simulink model "IEEE30_case"  (R2024b)
settings: Solver=FixedStepAuto  StartTime=0  StopTime=5  FixedStep=1e-7  RelTol=1e-3
values from neighbouring files (symbols this model uses):
  GFL_DFIG_7_C_bus = 0.08    [IEEE30_case_parameters.m]
  GFL_DFIG_7_D_mutual = 2.500000e+3    (= 2500)    [IEEE30_case_parameters.m]
  GFL_DFIG_7_f0 = 60    [IEEE30_case_parameters.m]
  GFL_DFIG_7_gPLLi = 3200    [IEEE30_case_parameters.m]
  GFL_DFIG_7_gPLLp = 650    [IEEE30_case_parameters.m]
  GFL_DFIG_7_H_WT = 0.4    [IEEE30_case_parameters.m]
  GFL_DFIG_7_Hg = 0.8    [IEEE30_case_parameters.m]
  GFL_DFIG_7_Igq_ref = 0    [IEEE30_case_parameters.m]
  GFL_DFIG_7_Ird_ref = 704.45696    [IEEE30_case_parameters.m]
  GFL_DFIG_7_KI_V = -300000    [IEEE30_case_parameters.m]
  GFL_DFIG_7_KP_V = -1000    [IEEE30_case_parameters.m]
  GFL_DFIG_7_Ksh = 1.254300e+4    (= 12543)    [IEEE30_case_parameters.m]
  GFL_DFIG_7_Lg = 0.000483    [IEEE30_case_parameters.m]
  GFL_DFIG_7_Lm_pu = 4    [IEEE30_case_parameters.m]
  GFL_DFIG_7_N = 100    [IEEE30_case_parameters.m]
  GFL_DFIG_7_p = 2    [IEEE30_case_parameters.m]
  GFL_DFIG_7_Pitch = 0    [IEEE30_case_parameters.m]
  GFL_DFIG_7_R = 44    [IEEE30_case_parameters.m]
  GFL_DFIG_7_Rg = 2.000000e-5    (= 2e-05)    [IEEE30_case_parameters.m]
  GFL_DFIG_7_rho = 1.225    [IEEE30_case_parameters.m]
  GFL_DFIG_7_rPLLi = 4500    [IEEE30_case_parameters.m]
  GFL_DFIG_7_rPLLp = 620    [IEEE30_case_parameters.m]
  GFL_DFIG_7_Rs_pu = 0.011    [IEEE30_case_parameters.m]
  GFL_DFIG_7_Sbase = 2.000000e+6    (= 2000000)    [IEEE30_case_parameters.m]
  GFL_DFIG_7_ugq_ref = 0    [IEEE30_case_parameters.m]
  GFL_DFIG_7_usd_ref = 0    [IEEE30_case_parameters.m]
  GFL_DFIG_7_Vbase = 690    [IEEE30_case_parameters.m]
  GFL_DFIG_7_Vdc_ref = 1200    [IEEE30_case_parameters.m]
  GFL_DFIG_7_wind = 12    [IEEE30_case_parameters.m]
  GFL_DFIG_7_wm_ref = 518.184209    [IEEE30_case_parameters.m]
  SG_D_13_D = 0.01056    [IEEE30_case_parameters.m]
  SG_D_13_EnableSaturation = 0    [IEEE30_case_parameters.m]
  SG_D_13_f0 = 60    [IEEE30_case_parameters.m]
  SG_D_13_H = 7.5    [IEEE30_case_parameters.m]
  SG_D_13_K_A = 20    [IEEE30_case_parameters.m]
  SG_D_13_K_E = 1.000000e+1    (= 10)    [IEEE30_case_parameters.m]
  SG_D_13_K_F = 2.363    [IEEE30_case_parameters.m]
  SG_D_13_K_s = 0.5    [IEEE30_case_parameters.m]
  SG_D_13_R_a = 0.001088    [IEEE30_case_parameters.m]
  SG_D_13_S_A = 1    [IEEE30_case_parameters.m]
  SG_D_13_S_B = 0.103    [IEEE30_case_parameters.m]
  SG_D_13_S_N = 10.659857    [IEEE30_case_parameters.m]
  SG_D_13_SpeedPara = 200    [IEEE30_case_parameters.m]
  SG_D_13_T_0 = 0.370163    [IEEE30_case_parameters.m]
  SG_D_13_T_1 = 0.3    [IEEE30_case_parameters.m]
  SG_D_13_T_2 = 0.05    [IEEE30_case_parameters.m]
  SG_D_13_T_3 = 0.02    [IEEE30_case_parameters.m]
  SG_D_13_T_4 = 0.005    [IEEE30_case_parameters.m]
  SG_D_13_T_A = 0.02    [IEEE30_case_parameters.m]
  SG_D_13_T_dd = 8.000000e+0    (= 8)    [IEEE30_case_parameters.m]
  SG_D_13_T_ddd = 0.04    [IEEE30_case_parameters.m]
  SG_D_13_T_E = 0.314    [IEEE30_case_parameters.m]
  SG_D_13_T_F = 0.35    [IEEE30_case_parameters.m]
  SG_D_13_T_qd = 0.8    [IEEE30_case_parameters.m]
  SG_D_13_T_qdd = 0.02    [IEEE30_case_parameters.m]
  SG_D_13_T_speed = 0.1    [IEEE30_case_parameters.m]
  SG_D_13_T_w = 0.5    [IEEE30_case_parameters.m]
  SG_D_13_V_ref = 1.696619    [IEEE30_case_parameters.m]
  SG_D_13_w_ref = 376.991118    [IEEE30_case_parameters.m]
  SG_D_13_x_d = 1.9    [IEEE30_case_parameters.m]
  SG_D_13_x_dd = 0.302    [IEEE30_case_parameters.m]
  SG_D_13_x_ddd = 0.204    [IEEE30_case_parameters.m]
  SG_D_13_x_l = 0.05    [IEEE30_case_parameters.m]
  SG_D_13_x_q = 1.3    [IEEE30_case_parameters.m]
  SG_D_13_x_qd = 0.5    [IEEE30_case_parameters.m]
  SG_D_13_x_qdd = 0.3    [IEEE30_case_parameters.m]
  SG_D_1_D = 0.01056    [IEEE30_case_parameters.m]
  SG_D_1_EnableSaturation = 0    [IEEE30_case_parameters.m]
  SG_D_1_f0 = 60    [IEEE30_case_parameters.m]
  SG_D_1_H = 7.5    [IEEE30_case_parameters.m]
  SG_D_1_K_A = 20    [IEEE30_case_parameters.m]
  SG_D_1_K_E = 1.000000e+1    (= 10)    [IEEE30_case_parameters.m]
  SG_D_1_K_F = 2.363    [IEEE30_case_parameters.m]
  SG_D_1_K_s = 0.5    [IEEE30_case_parameters.m]
  SG_D_1_R_a = 0.001088    [IEEE30_case_parameters.m]
  SG_D_1_S_A = 1    [IEEE30_case_parameters.m]
  SG_D_1_S_B = 0.103    [IEEE30_case_parameters.m]
  SG_D_1_S_N = 10.659857    [IEEE30_case_parameters.m]
  SG_D_1_SpeedPara = 200    [IEEE30_case_parameters.m]
  SG_D_1_T_0 = 0.259812    [IEEE30_case_parameters.m]
  SG_D_1_T_1 = 0.3    [IEEE30_case_parameters.m]
  SG_D_1_T_2 = 0.05    [IEEE30_case_parameters.m]
  SG_D_1_T_3 = 0.02    [IEEE30_case_parameters.m]
  SG_D_1_T_4 = 0.005    [IEEE30_case_parameters.m]
  SG_D_1_T_A = 0.02    [IEEE30_case_parameters.m]
  SG_D_1_T_dd = 8.000000e+0    (= 8)    [IEEE30_case_parameters.m]
  SG_D_1_T_ddd = 0.04    [IEEE30_case_parameters.m]
  SG_D_1_T_E = 0.314    [IEEE30_case_parameters.m]
  SG_D_1_T_F = 0.35    [IEEE30_case_parameters.m]
  SG_D_1_T_qd = 0.8    [IEEE30_case_parameters.m]
  SG_D_1_T_qdd = 0.02    [IEEE30_case_parameters.m]
  SG_D_1_T_speed = 0.1    [IEEE30_case_parameters.m]
  SG_D_1_T_w = 0.5    [IEEE30_case_parameters.m]
  SG_D_1_V_ref = 1.544107    [IEEE30_case_parameters.m]
  SG_D_1_w_ref = 376.991118    [IEEE30_case_parameters.m]
  SG_D_1_x_d = 1.9    [IEEE30_case_parameters.m]
  SG_D_1_x_dd = 0.302    [IEEE30_case_parameters.m]
  SG_D_1_x_ddd = 0.204    [IEEE30_case_parameters.m]
  SG_D_1_x_l = 0.05    [IEEE30_case_parameters.m]
  SG_D_1_x_q = 1.3    [IEEE30_case_parameters.m]
  SG_D_1_x_qd = 0.5    [IEEE30_case_parameters.m]
  SG_D_1_x_qdd = 0.3    [IEEE30_case_parameters.m]
  SG_D_22_D = 0.01056    [IEEE30_case_parameters.m]
  SG_D_22_EnableSaturation = 0    [IEEE30_case_parameters.m]
  SG_D_22_f0 = 60    [IEEE30_case_parameters.m]
  SG_D_22_H = 7.5    [IEEE30_case_parameters.m]
  SG_D_22_K_A = 20    [IEEE30_case_parameters.m]
  SG_D_22_K_E = 1.000000e+1    (= 10)    [IEEE30_case_parameters.m]
  SG_D_22_K_F = 2.363    [IEEE30_case_parameters.m]
  SG_D_22_K_s = 0.5    [IEEE30_case_parameters.m]
  SG_D_22_R_a = 0.001088    [IEEE30_case_parameters.m]
  SG_D_22_S_A = 1    [IEEE30_case_parameters.m]
  SG_D_22_S_B = 0.103    [IEEE30_case_parameters.m]
  SG_D_22_S_N = 10.659857    [IEEE30_case_parameters.m]
  SG_D_22_SpeedPara = 200    [IEEE30_case_parameters.m]
  SG_D_22_T_0 = 0.216121    [IEEE30_case_parameters.m]
  SG_D_22_T_1 = 0.3    [IEEE30_case_parameters.m]
  SG_D_22_T_2 = 0.05    [IEEE30_case_parameters.m]
  SG_D_22_T_3 = 0.02    [IEEE30_case_parameters.m]
  SG_D_22_T_4 = 0.005    [IEEE30_case_parameters.m]
  ... (+126 more)
(part 18 of 27)

== system IEEE30_case/SG_D_13/d_R_f_SG_D_13_block ==
  note: d_R_f_SG_D_13 in IEEE30_case
      | $-\frac{R_{f,\mathrm{SG},D,13}-\frac{E_{\mathrm{fd},\mathrm{SG},D,13}\,K_{F}}{T_{F}}}{T_{F}}$
      | Automatically generated on 2025-11-01 18:35:19 .
  State_E_fd_SG_D_13_3beb5 : Inport
  State_R_f_SG_D_13_66dca : Inport  Port=2
  Constant_K_F_6523e : Constant  Value=K_F
  Constant_T_F_407fc : Constant  Value=T_F
  Constant_T_F_fd8a5 : Constant  Value=T_F
  Divide_88de1 : Product  Inputs=*/
  Divide_8e027 : Product  Inputs=*/
  Product_33ef2 : Product
  Subtract_fc934 : Sum  Inputs=+-
  Blockout_d_R_f_SG_D_13_a8827 : Outport
  wires:
  State_E_fd_SG_D_13_3beb5/1 -> Product_33ef2/1
  Constant_K_F_6523e/1 -> Product_33ef2/2
  Product_33ef2/1 -> Divide_8e027/1
  Constant_T_F_fd8a5/1 -> Divide_88de1/2
  Divide_8e027/1 -> Subtract_fc934/1
  Constant_T_F_407fc/1 -> Divide_8e027/2
  State_R_f_SG_D_13_66dca/1 -> Subtract_fc934/2
  Subtract_fc934/1 -> Divide_88de1/1
  Divide_88de1/1 -> Blockout_d_R_f_SG_D_13_a8827/1

== system IEEE30_case/SG_D_13/d_T_m_SG_D_13_block ==
  note: d_T_m_SG_D_13 in IEEE30_case
      | $-\frac{T_{m,\mathrm{SG},D,13}-T_{0}+\frac{\mathrm{SpeedPara}\,\left(w_{\mathrm{SG},D,13}-w_{\mathrm{ref}}\right)}{2\,f_{0}\,\pi }}{T_{\mathrm{speed}}}$
      | Automatically generated on 2025-11-01 18:35:10 .
  State_w_SG_D_13_0a956 : Inport
  State_T_m_SG_D_13_e67bf : Inport  Port=2
  Add_0b399 : Sum
  Add_69f00 : Sum
  Constant_-1_245f6 : Constant  Value=-1
  Constant_2.0_2ba8d : Constant  Value=2.0
  Constant_SpeedPara_e01d4 : Constant  Value=SpeedPara
  Constant_T_0_5e408 : Constant  Value=T_0
  Constant_T_speed_48e6b : Constant  Value=T_speed
  Constant_f0_30e33 : Constant  Value=f0
  Constant_pi_c8119 : Constant  Value=pi
  Constant_w_ref_3479d : Constant  Value=w_ref
  Divide_6b714 : Product  Inputs=*/
  Divide_b8f6d : Product  Inputs=*/
  Product_17514 : Product
  Product_83a12 : Product
  Product_98a6e : Product
  Product_efe4b : Product
  Subtract_95fc6 : Sum  Inputs=+-
  Blockout_d_T_m_SG_D_13_01371 : Outport
  wires:
  Constant_SpeedPara_e01d4/1 -> Product_98a6e/1
  Constant_-1_245f6/1 -> Product_83a12/1
  State_w_SG_D_13_0a956/1 -> Product_83a12/2
  Constant_2.0_2ba8d/1 -> Product_efe4b/1
  Product_83a12/1 -> Add_0b399/1
  Constant_w_ref_3479d/1 -> Add_0b399/2
  Add_0b399/1 -> Product_98a6e/2
  Constant_pi_c8119/1 -> Product_efe4b/2
  Product_efe4b/1 -> Product_17514/1
  Constant_f0_30e33/1 -> Product_17514/2
  Product_98a6e/1 -> Divide_6b714/1
  Product_17514/1 -> Divide_6b714/2
  Divide_6b714/1 -> Add_69f00/1
  Constant_T_0_5e408/1 -> Add_69f00/2
  Constant_T_speed_48e6b/1 -> Divide_b8f6d/2
  Add_69f00/1 -> Subtract_95fc6/1
  State_T_m_SG_D_13_e67bf/1 -> Subtract_95fc6/2
  Subtract_95fc6/1 -> Divide_b8f6d/1
  Divide_b8f6d/1 -> Blockout_d_T_m_SG_D_13_01371/1

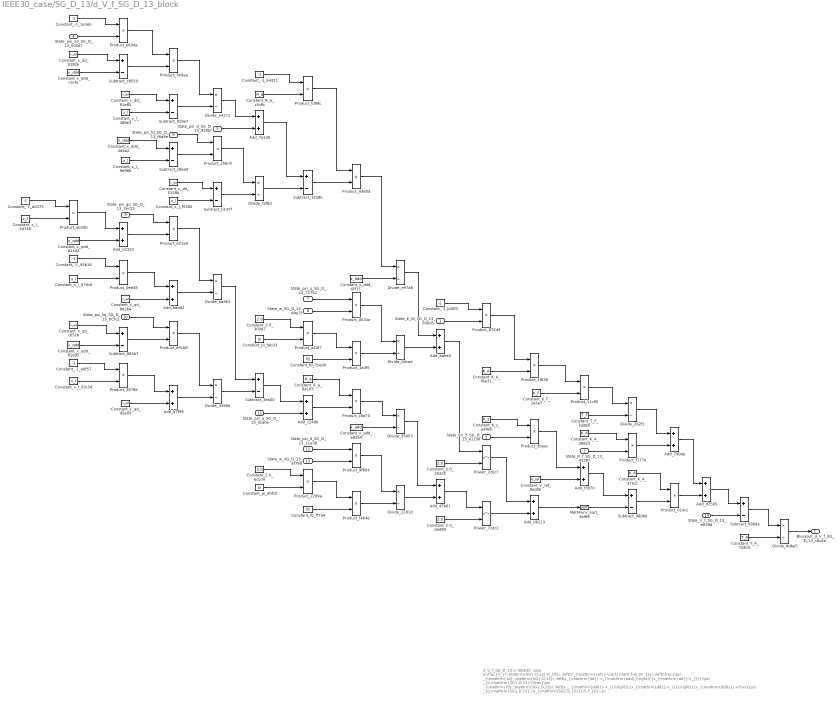
== system IEEE30_case/SG_D_13/d_V_f_SG_D_13_block ==
  note: d_V_f_SG_D_13 in IEEE30_case
      | $-\frac{V_{f,\mathrm{SG},D,13}-K_{A}\,\left(V_{\mathrm{ref}}-\sqrt{{\left(\frac{R_{a}\,\left(\frac{\psi _{\mathrm{1d},\mathrm{SG},D,13}\,\left(x_{\mathrm{dd}}-x_{\mathrm{ddd}}\right)}{x_{\mathrm{dd}}-x_{l}}-\psi _{d,\mathrm{SG},D,13}+\frac{\psi _{\mathrm{fd},\mathrm{SG},D,13}\,\left(x_{\mathrm{ddd}}-x_{l}\right)}{x_{\mathrm{dd}}-x_{l}}\right)}{x_{\mathrm{ddd}}}+\frac{\psi _{q,\mathrm{SG},D,13}\,w_{\mathrm{SG},D,13}}{2\,f_{0}\,\pi }\right)}^2+{\left(\frac{R_{a}\,\left(\psi _{q,\mathrm{SG},D,13}+\frac{\psi _{\mathrm{gq},\mathrm{SG},D,13}\,\left(x_{l}-x_{\mathrm{qdd}}\right)}{x_{l}-x_{\mathrm{qd}}}+\frac{\psi _{\mathrm{kq},\mathrm{SG},D,13}\,\left(x_{\mathrm{qd}}-x_{\mathrm{qdd}}\right)}{x_{l}-x_{\mathrm{qd}}}\right)}{x_{\mathrm{qdd}}}+\frac{\psi _{d,\mathrm{SG},D,13}\,w_{\mathrm{SG},D,13}}{2\,f_{0}\,\pi }\right)}^2}+K_{s}\,\mathrm{Px}_{3,\mathrm{SG},D,13}\right)-K_{A}\,R_{f,\mathrm{SG},D,13}+\frac{E_{\mathrm{fd},\mathrm{SG},D,13}\,K_{A}\,K_{F}}{T_{F}}}{T_{A}}$
      | Automatically generated on 2025-11-01 18:35:18 .
  State_E_fd_SG_D_13_836d5 : Inport
  State_R_f_SG_D_13_41787 : Inport  Port=2
  State_Px_3_SG_D_13_a1130 : Inport  Port=3
  State_psi_1d_SG_D_13_50567 : Inport  Port=4
  State_psi_d_SG_D_13_820bf : Inport  Port=5
  State_psi_fd_SG_D_13_f6a9e : Inport  Port=6
  State_psi_q_SG_D_13_72752 : Inport  Port=7
  State_w_SG_D_13_84e7f : Inport  Port=8
  State_psi_gq_SG_D_13_2ec25 : Inport  Port=9
  State_psi_kq_SG_D_13_bc5c2 : Inport  Port=10
  State_psi_q_SG_D_13_3ca0e : Inport  Port=11
  State_psi_d_SG_D_13_11e39 : Inport  Port=12
  State_w_SG_D_13_6f79b : Inport  Port=13
  State_V_f_SG_D_13_e839d : Inport  Port=14
  Add_06213 : Sum
  Add_47b61 : Sum
  Add_6add2 : Sum
  Add_790de : Sum
  Add_7a1d0 : Sum
  Add_aaea0 : Sum
  Add_b2152 : Sum
  Add_b7f99 : Sum
  Add_c24db : Sum
  Add_d25b5 : Sum
  Add_f3970 : Sum
  Constant_-1_1e3eb : Constant  Value=-1
  Constant_-1_54311 : Constant  Value=-1
  Constant_-1_94b18 : Constant  Value=-1
  Constant_-1_a0375 : Constant  Value=-1
  Constant_-1_b30f3 : Constant  Value=-1
  Constant_-1_e0f57 : Constant  Value=-1
  Constant_2.0_2b2c8 : Constant  Value=2.0
  Constant_2.0_303d7 : Constant  Value=2.0
  Constant_2.0_6cb7e : Constant  Value=2.0
  Constant_2.0_dad80 : Constant  Value=2.0
  Constant_K_A_28815 : Constant  Value=K_A
  Constant_K_A_375cc : Constant  Value=K_A
  Constant_K_A_f6e31 : Constant  Value=K_A
  Constant_K_F_2a5a7 : Constant  Value=K_F
  Constant_K_s_e4f69 : Constant  Value=K_s
  Constant_R_a_84103 : Constant  Value=R_a
  Constant_R_a_c5cfb : Constant  Value=R_a
  Constant_T_A_fd3bd : Constant  Value=T_A
  Constant_T_F_fdd58 : Constant  Value=T_F
  Constant_V_ref_8ad0b : Constant  Value=V_ref
  Constant_f0_7ced0 : Constant  Value=f0
  Constant_f0_ff7a4 : Constant  Value=f0
  Constant_pi_d0fc0 : Constant  Value=pi
  Constant_pi_fab33 : Constant  Value=pi
  Constant_x_dd_51586 : Constant  Value=x_dd
  Constant_x_dd_9182e : Constant  Value=x_dd
  Constant_x_dd_91e85 : Constant  Value=x_dd
  Constant_x_ddd_4d4a2 : Constant  Value=x_ddd
  Constant_x_ddd_6ff15 : Constant  Value=x_ddd
  Constant_x_ddd_c3cfa : Constant  Value=x_ddd
  Constant_x_l_03c5d : Constant  Value=x_l
  Constant_x_l_489e3 : Constant  Value=x_l
  Constant_x_l_5d748 : Constant  Value=x_l
  Constant_x_l_67dc6 : Constant  Value=x_l
  Constant_x_l_9e98b : Constant  Value=x_l
  Constant_x_l_f5300 : Constant  Value=x_l
  Constant_x_qd_862b4 : Constant  Value=x_qd
  Constant_x_qd_c05cb : Constant  Value=x_qd
  Constant_x_qd_d2e03 : Constant  Value=x_qd
  Constant_x_qdd_81a95 : Constant  Value=x_qdd
  Constant_x_qdd_a14d2 : Constant  Value=x_qdd
  Constant_x_qdd_a82a4 : Constant  Value=x_qdd
  Divide_0dcae : Product  Inputs=*/
  Divide_2201d : Product  Inputs=*/
  Divide_262f1 : Product  Inputs=*/
  Divide_35053 : Product  Inputs=*/
  Divide_4398e : Product  Inputs=*/
  Divide_8dbe5 : Product  Inputs=*/
  Divide_aa963 : Product  Inputs=*/
  Divide_e4271 : Product  Inputs=*/
  Divide_e97a6 : Product  Inputs=*/
  Divide_faf8d : Product  Inputs=*/
  MathFunc_sqrt_3a9f8 : Sqrt
  Power_2c6c7 : Math  Operator=pow
  Power_7cdc2 : Math  Operator=pow
  Product_014cc : Product
  Product_0ee38 : Product
  Product_11c85 : Product
  Product_1a3f5 : Product
  Product_1f638 : Product
  Product_2299a : Product
  Product_256c9 : Product
  Product_3978e : Product
  Product_3beec : Product
  Product_3e9ea : Product
  Product_872d3 : Product
  Product_93e0d : Product
  Product_9f804 : Product
  Product_a13f7 : Product
  Product_ab3db : Product
  Product_b634a : Product
  Product_c8a70 : Product
  Product_d534a : Product
  Product_e21a9 : Product
  Product_e91b8 : Product
  Product_f177e : Product
  Product_f464e : Product
  Product_fd99c : Product
  Subtract_096da : Sum  Inputs=+-
  Subtract_3228b : Sum  Inputs=+-
  Subtract_3ea00 : Sum  Inputs=+-
  Subtract_883b7 : Sum  Inputs=+-
  Subtract_919e7 : Sum  Inputs=+-
  Subtract_b147f : Sum  Inputs=+-
  Subtract_c8550 : Sum  Inputs=+-
  Subtract_c8ed4 : Sum  Inputs=+-
  Subtract_d60bd : Sum  Inputs=+-
  Blockout_d_V_f_SG_D_13_c6c4a : Outport
  wires:
  Add_d25b5/1 -> Subtract_096da/1
  Product_3978e/1 -> Add_b7f99/1
  Constant_-1_e0f57/1 -> Product_3978e/1
  Constant_x_qdd_a14d2/1 -> Add_b2152/2
  Constant_x_qd_d2e03/1 -> Add_b7f99/2
  Constant_-1_a0375/1 -> Product_ab3db/1
  Product_ab3db/1 -> Add_b2152/1
  Constant_x_ddd_c3cfa/1 -> Subtract_c8550/2
  Product_fd99c/1 -> Product_93e0d/1
  Add_b7f99/1 -> Divide_4398e/2
  Constant_-1_54311/1 -> Product_fd99c/1
  Constant_x_l_5d748/1 -> Product_ab3db/2
  Divide_2201d/1 -> Add_47b61/2
  Product_b634a/1 -> Product_3e9ea/1
  Constant_-1_1e3eb/1 -> Product_b634a/1
  Constant_x_qd_862b4/1 -> Add_6add2/2
  Subtract_c8550/1 -> Product_3e9ea/2
  Constant_x_dd_9182e/1 -> Subtract_c8550/1
  Divide_4398e/1 -> Subtract_3ea00/2
  State_psi_1d_SG_D_13_50567/1 -> Product_b634a/2
  Constant_-1_94b18/1 -> Product_0ee38/1
  State_psi_q_SG_D_13_3ca0e/1 -> Add_c24db/2
  Product_0ee38/1 -> Add_6add2/1
  Divide_e4271/1 -> Add_7a1d0/1
  Constant_x_l_67dc6/1 -> Product_0ee38/2
  Subtract_883b7/1 -> Product_e91b8/2
  State_psi_d_SG_D_13_820bf/1 -> Add_7a1d0/2
  Constant_x_qd_c05cb/1 -> Subtract_883b7/1
  Constant_x_qdd_81a95/1 -> Subtract_883b7/2
  Add_b2152/1 -> Product_e21a9/2
  Constant_x_l_03c5d/1 -> Product_3978e/2
  Constant_2.0_6cb7e/1 -> Product_2299a/1
  Subtract_919e7/1 -> Divide_e4271/2
  Constant_x_dd_91e85/1 -> Subtract_919e7/1
  Constant_pi_d0fc0/1 -> Product_2299a/2
  Constant_x_l_489e3/1 -> Subtract_919e7/2
  Subtract_c8ed4/1 -> Product_256c9/2
  Divide_262f1/1 -> Add_790de/1
  Constant_x_ddd_4d4a2/1 -> Subtract_c8ed4/1
  Constant_x_l_9e98b/1 -> Subtract_c8ed4/2
  Product_e21a9/1 -> Divide_aa963/1
  State_psi_gq_SG_D_13_2ec25/1 -> Product_e21a9/1
  Product_e91b8/1 -> Divide_4398e/1
  State_psi_kq_SG_D_13_bc5c2/1 -> Product_e91b8/1
  Product_3e9ea/1 -> Divide_e4271/1
  Product_256c9/1 -> Divide_faf8d/1
  State_psi_fd_SG_D_13_f6a9e/1 -> Product_256c9/1
  Subtract_b147f/1 -> Divide_faf8d/2
  Constant_x_dd_51586/1 -> Subtract_b147f/1
  Constant_x_l_f5300/1 -> Subtract_b147f/2
  Add_6add2/1 -> Divide_aa963/2
  Divide_aa963/1 -> Subtract_3ea00/1
  Constant_R_a_c5cfb/1 -> Product_fd99c/2
  Add_7a1d0/1 -> Subtract_3228b/1
  Constant_f0_7ced0/1 -> Product_1a3f5/2
  Divide_faf8d/1 -> Subtract_3228b/2
  Product_a13f7/1 -> Product_1a3f5/1
  Constant_2.0_303d7/1 -> Product_a13f7/1
  Constant_pi_fab33/1 -> Product_a13f7/2
  State_w_SG_D_13_84e7f/1 -> Product_d534a/2
  Subtract_3ea00/1 -> Add_c24db/1
  Subtract_3228b/1 -> Product_93e0d/2
  State_psi_q_SG_D_13_72752/1 -> Product_d534a/1
  Constant_R_a_84103/1 -> Product_c8a70/1
  Add_c24db/1 -> Product_c8a70/2
  State_psi_d_SG_D_13_11e39/1 -> Product_9f804/1
  State_w_SG_D_13_6f79b/1 -> Product_9f804/2
  Product_2299a/1 -> Product_f464e/1
  Constant_f0_ff7a4/1 -> Product_f464e/2
  Product_93e0d/1 -> Divide_e97a6/1
  Constant_x_ddd_6ff15/1 -> Divide_e97a6/2
  Product_d534a/1 -> Divide_0dcae/1
  Product_1a3f5/1 -> Divide_0dcae/2
  Product_c8a70/1 -> Divide_35053/1
  Constant_x_qdd_a82a4/1 -> Divide_35053/2
  Product_9f804/1 -> Divide_2201d/1
  Product_f464e/1 -> Divide_2201d/2
  Divide_e97a6/1 -> Add_aaea0/1
  Divide_0dcae/1 -> Add_aaea0/2
  Divide_35053/1 -> Add_47b61/1
  Constant_-1_b30f3/1 -> Product_872d3/1
  State_E_fd_SG_D_13_836d5/1 -> Product_872d3/2
  Add_aaea0/1 -> Power_2c6c7/1
  Constant_2.0_2b2c8/1 -> Power_2c6c7/2
  Add_47b61/1 -> Power_7cdc2/1
  Constant_2.0_dad80/1 -> Power_7cdc2/2
  Product_872d3/1 -> Product_1f638/1
  Constant_K_A_f6e31/1 -> Product_1f638/2
  Constant_K_s_e4f69/1 -> Product_3beec/1
  State_Px_3_SG_D_13_a1130/1 -> Product_3beec/2
  Power_2c6c7/1 -> Add_06213/1
  Power_7cdc2/1 -> Add_06213/2
  Product_1f638/1 -> Product_11c85/1
  Constant_K_F_2a5a7/1 -> Product_11c85/2
  Product_3beec/1 -> Add_f3970/1
  Constant_V_ref_8ad0b/1 -> Add_f3970/2
  Add_06213/1 -> MathFunc_sqrt_3a9f8/1
  Product_11c85/1 -> Divide_262f1/1
  Constant_T_F_fdd58/1 -> Divide_262f1/2
  Constant_K_A_28815/1 -> Product_f177e/1
  State_R_f_SG_D_13_41787/1 -> Product_f177e/2
  Add_f3970/1 -> Subtract_d60bd/1
  MathFunc_sqrt_3a9f8/1 -> Subtract_d60bd/2
  Product_f177e/1 -> Add_790de/2
  Constant_K_A_375cc/1 -> Product_014cc/1
  Subtract_d60bd/1 -> Product_014cc/2
  Add_790de/1 -> Add_d25b5/1
  Product_014cc/1 -> Add_d25b5/2
  State_V_f_SG_D_13_e839d/1 -> Subtract_096da/2
  Subtract_096da/1 -> Divide_8dbe5/1
  Constant_T_A_fd3bd/1 -> Divide_8dbe5/2
  Divide_8dbe5/1 -> Blockout_d_V_f_SG_D_13_c6c4a/1

== system IEEE30_case/SG_D_13/d_psi_1d_SG_D_13_block ==
  note: d_psi_1d_SG_D_13 in IEEE30_case
      | $-\frac{\psi _{\mathrm{1d},\mathrm{SG},D,13}-\psi _{\mathrm{fd},\mathrm{SG},D,13}+\frac{\left(x_{\mathrm{dd}}-x_{l}\right)\,\left(\frac{\psi _{\mathrm{1d},\mathrm{SG},D,13}\,\left(x_{\mathrm{dd}}-x_{\mathrm{ddd}}\right)}{x_{\mathrm{dd}}-x_{l}}-\psi _{d,\mathrm{SG},D,13}+\frac{\psi _{\mathrm{fd},\mathrm{SG},D,13}\,\left(x_{\mathrm{ddd}}-x_{l}\right)}{x_{\mathrm{dd}}-x_{l}}\right)}{x_{\mathrm{ddd}}}}{T_{\mathrm{ddd}}}$
      | Automatically generated on 2025-11-01 18:34:53 .
  State_psi_1d_SG_D_13_5ea9c : Inport
  State_psi_fd_SG_D_13_02d25 : Inport  Port=2
  State_psi_1d_SG_D_13_b86a3 : Inport  Port=3
  State_psi_d_SG_D_13_069ec : Inport  Port=4
  State_psi_fd_SG_D_13_cf913 : Inport  Port=5
  Add_64976 : Sum
  Add_d8aae : Sum
  Add_f903f : Sum
  Constant_-1_6ab43 : Constant  Value=-1
  Constant_-1_94687 : Constant  Value=-1
  Constant_T_ddd_f7478 : Constant  Value=T_ddd
  Constant_x_dd_4d6bb : Constant  Value=x_dd
  Constant_x_dd_80146 : Constant  Value=x_dd
  Constant_x_dd_f3c0c : Constant  Value=x_dd
  Constant_x_dd_f7df2 : Constant  Value=x_dd
  Constant_x_ddd_219b0 : Constant  Value=x_ddd
  Constant_x_ddd_6a218 : Constant  Value=x_ddd
  Constant_x_ddd_9b8b1 : Constant  Value=x_ddd
  Constant_x_l_00293 : Constant  Value=x_l
  Constant_x_l_80933 : Constant  Value=x_l
  Constant_x_l_8fdb8 : Constant  Value=x_l
  Constant_x_l_be718 : Constant  Value=x_l
  Divide_7ef31 : Product  Inputs=*/
  Divide_84808 : Product  Inputs=*/
  Divide_cdf31 : Product  Inputs=*/
  Divide_e7112 : Product  Inputs=*/
  Product_4bf29 : Product
  Product_b6823 : Product
  Product_c120e : Product
  Product_e6d69 : Product
  Product_feeb6 : Product
  Subtract_0a55e : Sum  Inputs=+-
  Subtract_0b047 : Sum  Inputs=+-
  Subtract_434d9 : Sum  Inputs=+-
  Subtract_a0698 : Sum  Inputs=+-
  Subtract_afe7a : Sum  Inputs=+-
  Subtract_f4760 : Sum  Inputs=+-
  Blockout_d_psi_1d_SG_D_13_abf30 : Outport
  wires:
  Constant_-1_6ab43/1 -> Product_e6d69/1
  Divide_84808/1 -> Subtract_0a55e/2
  Constant_x_ddd_6a218/1 -> Subtract_434d9/2
  State_psi_1d_SG_D_13_b86a3/1 -> Product_e6d69/2
  Add_d8aae/1 -> Subtract_0a55e/1
  Product_e6d69/1 -> Product_feeb6/1
  Constant_x_dd_f7df2/1 -> Subtract_434d9/1
  Subtract_434d9/1 -> Product_feeb6/2
  State_psi_d_SG_D_13_069ec/1 -> Add_d8aae/2
  Subtract_0b047/1 -> Divide_e7112/2
  Constant_x_dd_80146/1 -> Subtract_0b047/1
  Constant_x_l_be718/1 -> Subtract_0b047/2
  Subtract_afe7a/1 -> Product_4bf29/2
  Constant_x_ddd_9b8b1/1 -> Subtract_afe7a/1
  Add_f903f/1 -> Divide_7ef31/1
  Constant_x_l_00293/1 -> Subtract_afe7a/2
  State_psi_fd_SG_D_13_02d25/1 -> Add_64976/2
  Product_feeb6/1 -> Divide_e7112/1
  Product_4bf29/1 -> Divide_84808/1
  State_psi_fd_SG_D_13_cf913/1 -> Product_4bf29/1
  Subtract_a0698/1 -> Divide_84808/2
  Constant_x_dd_f3c0c/1 -> Subtract_a0698/1
  Constant_x_l_8fdb8/1 -> Subtract_a0698/2
  Divide_e7112/1 -> Add_d8aae/1
  Constant_x_dd_4d6bb/1 -> Subtract_f4760/1
  Constant_x_l_80933/1 -> Subtract_f4760/2
  Constant_-1_94687/1 -> Product_c120e/1
  State_psi_1d_SG_D_13_5ea9c/1 -> Product_c120e/2
  Subtract_f4760/1 -> Product_b6823/1
  Divide_cdf31/1 -> Add_f903f/2
  Subtract_0a55e/1 -> Product_b6823/2
  Product_c120e/1 -> Add_64976/1
  Product_b6823/1 -> Divide_cdf31/1
  Constant_x_ddd_219b0/1 -> Divide_cdf31/2
  Add_64976/1 -> Add_f903f/1
  Divide_7ef31/1 -> Blockout_d_psi_1d_SG_D_13_abf30/1
  Constant_T_ddd_f7478/1 -> Divide_7ef31/2

== system IEEE30_case/SG_D_13/d_psi_d_SG_D_13_block ==
  note: d_psi_d_SG_D_13 in IEEE30_case
      | $2\,\pi \,f_{0}\,\left(v_{d,\mathrm{SG},D,13}\,\sin\left(\theta _{\mathrm{SG},D,13}\right)-v_{q,\mathrm{SG},D,13}\,\cos\left(\theta _{\mathrm{SG},D,13}\right)+\frac{R_{a}\,\left(\frac{\psi _{\mathrm{1d},\mathrm{SG},D,13}\,\left(x_{\mathrm{dd}}-x_{\mathrm{ddd}}\right)}{x_{\mathrm{dd}}-x_{l}}-\psi _{d,\mathrm{SG},D,13}+\frac{\psi _{\mathrm{fd},\mathrm{SG},D,13}\,\left(x_{\mathrm{ddd}}-x_{l}\right)}{x_{\mathrm{dd}}-x_{l}}\right)}{x_{\mathrm{ddd}}}+\frac{\psi _{q,\mathrm{SG},D,13}\,w_{\mathrm{SG},D,13}}{2\,f_{0}\,\pi }\right)$
      | Automatically generated on 2025-11-01 18:34:43 .
  State_psi_1d_SG_D_13_9b112 : Inport
  State_psi_d_SG_D_13_8aacd : Inport  Port=2
  State_psi_fd_SG_D_13_f7d01 : Inport  Port=3
  Input_v_d_SG_D_13_b2974 : Inport  Port=4
  State_theta_SG_D_13_2e399 : Inport  Port=5
  Input_v_q_SG_D_13_58b42 : Inport  Port=6
  State_theta_SG_D_13_2b5b0 : Inport  Port=7
  State_psi_q_SG_D_13_c4468 : Inport  Port=8
  State_w_SG_D_13_602e4 : Inport  Port=9
  Add_29685 : Sum
  Add_2c7a8 : Sum
  Constant_-1_027db : Constant  Value=-1
  Constant_-2.0_89d97 : Constant  Value=-2.0
  Constant_2.0_b9a2b : Constant  Value=2.0
  Constant_R_a_ac41c : Constant  Value=R_a
  Constant_f0_1ac44 : Constant  Value=f0
  Constant_f0_7e92a : Constant  Value=f0
  Constant_pi_14aa3 : Constant  Value=pi
  Constant_pi_c7930 : Constant  Value=pi
  Constant_x_dd_52491 : Constant  Value=x_dd
  Constant_x_dd_676dc : Constant  Value=x_dd
  Constant_x_dd_a3984 : Constant  Value=x_dd
  Constant_x_ddd_59ebf : Constant  Value=x_ddd
  Constant_x_ddd_b72d8 : Constant  Value=x_ddd
  Constant_x_ddd_e123d : Constant  Value=x_ddd
  Constant_x_l_0810d : Constant  Value=x_l
  Constant_x_l_2d304 : Constant  Value=x_l
  Constant_x_l_a4cda : Constant  Value=x_l
  Divide_32eb9 : Product  Inputs=*/
  Divide_51be6 : Product  Inputs=*/
  Divide_eb74c : Product  Inputs=*/
  Divide_f6f2b : Product  Inputs=*/
  MathFunc_cos_8365f : Trigonometry  Operator=cos
  MathFunc_sin_b73cc : Trigonometry
  Product_07adc : Product
  Product_1f085 : Product
  Product_37a6e : Product
  Product_74875 : Product
  Product_a0afa : Product
  Product_b904d : Product
  Product_c9348 : Product
  Product_d3610 : Product
  Product_dd4f5 : Product
  Product_ddecb : Product
  Product_e7fe1 : Product
  Product_fa288 : Product
  Subtract_03d8f : Sum  Inputs=+-
  Subtract_6d1e1 : Sum  Inputs=+-
  Subtract_72d5f : Sum  Inputs=+-
  Subtract_877e5 : Sum  Inputs=+-
  Subtract_8b26f : Sum  Inputs=+-
  Subtract_92122 : Sum  Inputs=+-
  Subtract_945ec : Sum  Inputs=+-
  Blockout_d_psi_d_SG_D_13_069d2 : Outport
  wires:
  Constant_-1_027db/1 -> Product_e7fe1/1
  Product_e7fe1/1 -> Product_ddecb/1
  Add_29685/1 -> Subtract_877e5/1
  State_psi_1d_SG_D_13_9b112/1 -> Product_e7fe1/2
  Constant_x_dd_a3984/1 -> Subtract_8b26f/1
  Constant_f0_1ac44/1 -> Product_d3610/2
  Constant_x_dd_676dc/1 -> Subtract_945ec/1
  Subtract_877e5/1 -> Product_07adc/2
  Constant_x_ddd_59ebf/1 -> Subtract_8b26f/2
  Subtract_8b26f/1 -> Product_ddecb/2
  Constant_x_l_0810d/1 -> Subtract_945ec/2
  Subtract_03d8f/1 -> Product_74875/2
  Constant_x_ddd_b72d8/1 -> Subtract_03d8f/1
  Constant_x_l_a4cda/1 -> Subtract_03d8f/2
  Product_ddecb/1 -> Divide_51be6/1
  Constant_pi_14aa3/1 -> Product_1f085/2
  Subtract_945ec/1 -> Divide_51be6/2
  Product_74875/1 -> Divide_32eb9/1
  State_psi_fd_SG_D_13_f7d01/1 -> Product_74875/1
  Subtract_92122/1 -> Divide_32eb9/2
  Constant_x_dd_52491/1 -> Subtract_92122/1
  Constant_x_l_2d304/1 -> Subtract_92122/2
  Divide_51be6/1 -> Add_2c7a8/1
  Product_1f085/1 -> Product_d3610/1
  Constant_-2.0_89d97/1 -> Product_1f085/1
  State_psi_d_SG_D_13_8aacd/1 -> Add_2c7a8/2
  Add_2c7a8/1 -> Subtract_72d5f/1
  State_w_SG_D_13_602e4/1 -> Product_fa288/2
  Divide_32eb9/1 -> Subtract_72d5f/2
  Product_37a6e/1 -> Divide_eb74c/1
  Constant_R_a_ac41c/1 -> Product_37a6e/1
  Subtract_72d5f/1 -> Product_37a6e/2
  Constant_pi_c7930/1 -> Product_c9348/2
  MathFunc_sin_b73cc/1 -> Product_a0afa/2
  State_theta_SG_D_13_2e399/1 -> MathFunc_sin_b73cc/1
  Constant_x_ddd_e123d/1 -> Divide_eb74c/2
  Product_d3610/1 -> Product_07adc/1
  Input_v_d_SG_D_13_b2974/1 -> Product_a0afa/1
  State_theta_SG_D_13_2b5b0/1 -> MathFunc_cos_8365f/1
  Constant_2.0_b9a2b/1 -> Product_c9348/1
  Divide_eb74c/1 -> Subtract_6d1e1/1
  Product_a0afa/1 -> Subtract_6d1e1/2
  Product_b904d/1 -> Add_29685/2
  Input_v_q_SG_D_13_58b42/1 -> Product_b904d/1
  MathFunc_cos_8365f/1 -> Product_b904d/2
  State_psi_q_SG_D_13_c4468/1 -> Product_fa288/1
  Product_c9348/1 -> Product_dd4f5/1
  Constant_f0_7e92a/1 -> Product_dd4f5/2
  Subtract_6d1e1/1 -> Add_29685/1
  Product_fa288/1 -> Divide_f6f2b/1
  Product_dd4f5/1 -> Divide_f6f2b/2
  Divide_f6f2b/1 -> Subtract_877e5/2
  Product_07adc/1 -> Blockout_d_psi_d_SG_D_13_069d2/1

== system IEEE30_case/SG_D_13/d_psi_fd_SG_D_13_block ==
  note: d_psi_fd_SG_D_13 in IEEE30_case
      | $-\frac{\psi _{\mathrm{fd},\mathrm{SG},D,13}-E_{\mathrm{fd},\mathrm{SG},D,13}+\left(x_{d}-x_{\mathrm{dd}}\right)\,\left(\frac{\frac{\psi _{\mathrm{1d},\mathrm{SG},D,13}\,\left(x_{\mathrm{dd}}-x_{\mathrm{ddd}}\right)}{x_{\mathrm{dd}}-x_{l}}-\psi _{d,\mathrm{SG},D,13}+\frac{\psi _{\mathrm{fd},\mathrm{SG},D,13}\,\left(x_{\mathrm{ddd}}-x_{l}\right)}{x_{\mathrm{dd}}-x_{l}}}{x_{\mathrm{ddd}}}-\frac{\left(x_{\mathrm{dd}}-x_{\mathrm{ddd}}\right)\,\left(\psi _{\mathrm{1d},\mathrm{SG},D,13}-\psi _{\mathrm{fd},\mathrm{SG},D,13}+\frac{\left(x_{\mathrm{dd}}-x_{l}\right)\,\left(\frac{\psi _{\mathrm{1d},\mathrm{SG},D,13}\,\left(x_{\mathrm{dd}}-x_{\mathrm{ddd}}\right)}{x_{\mathrm{dd}}-x_{l}}-\psi _{d,\mathrm{SG},D,13}+\frac{\psi _{\mathrm{fd},\mathrm{SG},D,13}\,\left(x_{\mathrm{ddd}}-x_{l}\right)}{x_{\mathrm{dd}}-x_{l}}\right)}{x_{\mathrm{ddd}}}\right)}{{\left(x_{\mathrm{dd}}-x_{l}\right)}^2}\right)}{T_{\mathrm{dd}}}$
      | Automatically generated on 2025-11-01 18:34:51 .
  State_E_fd_SG_D_13_51a5d : Inport
  State_psi_fd_SG_D_13_37be0 : Inport  Port=2
  State_psi_1d_SG_D_13_e35eb : Inport  Port=3
  State_psi_fd_SG_D_13_e705d : Inport  Port=4
  State_psi_1d_SG_D_13_2bb65 : Inport  Port=5
  State_psi_d_SG_D_13_f5341 : Inport  Port=6
  State_psi_fd_SG_D_13_f9d12 : Inport  Port=7
  State_psi_1d_SG_D_13_4aa56 : Inport  Port=8
  State_psi_d_SG_D_13_8fa6c : Inport  Port=9
  State_psi_fd_SG_D_13_a6df8 : Inport  Port=10
  Add_82cd2 : Sum
  Add_9010e : Sum
  Constant_-1_97f3b : Constant  Value=-1
  Constant_-1_b7293 : Constant  Value=-1
  Constant_-1_e7324 : Constant  Value=-1
  Constant_2.0_317ba : Constant  Value=2.0
  Constant_T_dd_788cd : Constant  Value=T_dd
  Constant_x_d_b5ef4 : Constant  Value=x_d
  Constant_x_dd_00560 : Constant  Value=x_dd
  Constant_x_dd_19cec : Constant  Value=x_dd
  Constant_x_dd_254af : Constant  Value=x_dd
  Constant_x_dd_25536 : Constant  Value=x_dd
  Constant_x_dd_525f7 : Constant  Value=x_dd
  Constant_x_dd_796be : Constant  Value=x_dd
  Constant_x_dd_8482f : Constant  Value=x_dd
  Constant_x_dd_8c97f : Constant  Value=x_dd
  Constant_x_dd_e8a85 : Constant  Value=x_dd
  Constant_x_dd_ed741 : Constant  Value=x_dd
  Constant_x_ddd_1d9c2 : Constant  Value=x_ddd
  Constant_x_ddd_307b0 : Constant  Value=x_ddd
  Constant_x_ddd_735ff : Constant  Value=x_ddd
  Constant_x_ddd_758b5 : Constant  Value=x_ddd
  Constant_x_ddd_7fa27 : Constant  Value=x_ddd
  Constant_x_ddd_89921 : Constant  Value=x_ddd
  Constant_x_ddd_caf9c : Constant  Value=x_ddd
  Constant_x_l_0dde2 : Constant  Value=x_l
  Constant_x_l_1e6eb : Constant  Value=x_l
  Constant_x_l_2120d : Constant  Value=x_l
  Constant_x_l_54d7b : Constant  Value=x_l
  Constant_x_l_7993c : Constant  Value=x_l
  Constant_x_l_9adb5 : Constant  Value=x_l
  Constant_x_l_b67f7 : Constant  Value=x_l
  Constant_x_l_e8ff2 : Constant  Value=x_l
  Divide_32964 : Product  Inputs=*/
  Divide_505fe : Product  Inputs=*/
  Divide_53926 : Product  Inputs=*/
  Divide_a2d80 : Product  Inputs=*/
  Divide_a7c1a : Product  Inputs=*/
  Divide_c7856 : Product  Inputs=*/
  Divide_d9d2a : Product  Inputs=*/
  Divide_e738d : Product  Inputs=*/
  Power_d7519 : Math  Operator=pow
  Product_01015 : Product
  Product_1da9b : Product
  Product_30149 : Product
  Product_5f7b4 : Product
  Product_6c0af : Product
  Product_8a056 : Product
  Product_934a9 : Product
  Product_a5637 : Product
  Product_c12ba : Product
  Product_c378b : Product
  Subtract_01dfc : Sum  Inputs=+-
  Subtract_1b8ec : Sum  Inputs=+-
  Subtract_1eca1 : Sum  Inputs=+-
  Subtract_2704a : Sum  Inputs=+-
  Subtract_27118 : Sum  Inputs=+-
  Subtract_4d422 : Sum  Inputs=+-
  Subtract_4fed6 : Sum  Inputs=+-
  Subtract_50e9d : Sum  Inputs=+-
  Subtract_56b16 : Sum  Inputs=+-
  Subtract_68bad : Sum  Inputs=+-
  Subtract_744ea : Sum  Inputs=+-
  Subtract_7c9b3 : Sum  Inputs=+-
  Subtract_9b871 : Sum  Inputs=+-
  Subtract_a10ba : Sum  Inputs=+-
  Subtract_a14fc : Sum  Inputs=+-
  Subtract_bb3d2 : Sum  Inputs=+-
  Subtract_c4390 : Sum  Inputs=+-
  Subtract_cbd76 : Sum  Inputs=+-
  Subtract_e9930 : Sum  Inputs=+-
  Blockout_d_psi_fd_SG_D_13_87f69 : Outport
  wires:
  Constant_x_l_54d7b/1 -> Subtract_a14fc/2
  Constant_-1_b7293/1 -> Product_8a056/1
  Product_8a056/1 -> Product_01015/1
  Constant_x_dd_ed741/1 -> Subtract_a10ba/1
  Subtract_a10ba/1 -> Product_01015/2
  State_psi_1d_SG_D_13_2bb65/1 -> Product_8a056/2
  Subtract_bb3d2/1 -> Divide_a7c1a/2
  Constant_x_dd_254af/1 -> Subtract_bb3d2/1
  Constant_x_ddd_735ff/1 -> Subtract_a10ba/2
  Constant_x_l_7993c/1 -> Subtract_bb3d2/2
  Subtract_4fed6/1 -> Product_6c0af/2
  Constant_x_ddd_758b5/1 -> Subtract_4fed6/1
  Constant_x_l_0dde2/1 -> Subtract_4fed6/2
  Product_01015/1 -> Divide_a7c1a/1
  Product_6c0af/1 -> Divide_a2d80/1
  Constant_x_l_b67f7/1 -> Subtract_e9930/2
  State_E_fd_SG_D_13_51a5d/1 -> Subtract_c4390/1
  State_psi_fd_SG_D_13_f9d12/1 -> Product_6c0af/1
  Subtract_1b8ec/1 -> Product_a5637/1
  Subtract_e9930/1 -> Divide_a2d80/2
  Constant_x_dd_8c97f/1 -> Subtract_e9930/1
  Divide_a7c1a/1 -> Add_9010e/1
  State_psi_d_SG_D_13_f5341/1 -> Add_9010e/2
  Subtract_a14fc/1 -> Product_1da9b/1
  Constant_x_dd_00560/1 -> Subtract_a14fc/1
  Add_9010e/1 -> Subtract_744ea/1
  Divide_a2d80/1 -> Subtract_744ea/2
  Product_c12ba/1 -> Product_30149/1
  Constant_-1_e7324/1 -> Product_c12ba/1
  State_psi_1d_SG_D_13_4aa56/1 -> Product_c12ba/2
  Constant_2.0_317ba/1 -> Power_d7519/2
  Subtract_68bad/1 -> Product_30149/2
  Constant_x_dd_e8a85/1 -> Subtract_68bad/1
  Constant_x_ddd_89921/1 -> Subtract_68bad/2
  Subtract_744ea/1 -> Product_1da9b/2
  Constant_x_l_1e6eb/1 -> Subtract_27118/2
  Subtract_cbd76/1 -> Divide_32964/2
  Constant_x_dd_25536/1 -> Subtract_cbd76/1
  Subtract_50e9d/1 -> Subtract_01dfc/1
  State_psi_1d_SG_D_13_e35eb/1 -> Subtract_50e9d/1
  Constant_x_l_9adb5/1 -> Subtract_cbd76/2
  Constant_x_ddd_7fa27/1 -> Subtract_9b871/1
  Subtract_4d422/1 -> Divide_53926/2
  Constant_x_l_2120d/1 -> Subtract_9b871/2
  Constant_x_dd_525f7/1 -> Subtract_4d422/1
  Product_5f7b4/1 -> Product_934a9/1
  Subtract_1eca1/1 -> Product_5f7b4/2
  Constant_x_dd_796be/1 -> Subtract_1eca1/1
  State_psi_fd_SG_D_13_a6df8/1 -> Product_c378b/1
  Constant_x_ddd_307b0/1 -> Subtract_1eca1/2
  State_psi_fd_SG_D_13_e705d/1 -> Subtract_50e9d/2
  Product_1da9b/1 -> Divide_c7856/1
  Constant_x_ddd_1d9c2/1 -> Divide_c7856/2
  Product_30149/1 -> Divide_32964/1
  Subtract_9b871/1 -> Product_c378b/2
  Product_c378b/1 -> Divide_53926/1
  Constant_x_l_e8ff2/1 -> Subtract_4d422/2
  Constant_-1_97f3b/1 -> Product_5f7b4/1
  Divide_32964/1 -> Add_82cd2/1
  Divide_c7856/1 -> Subtract_01dfc/2
  Subtract_27118/1 -> Power_d7519/1
  Constant_x_dd_19cec/1 -> Subtract_27118/1
  State_psi_d_SG_D_13_8fa6c/1 -> Add_82cd2/2
  Subtract_01dfc/1 -> Product_934a9/2
  Add_82cd2/1 -> Subtract_56b16/1
  Divide_53926/1 -> Subtract_56b16/2
  Product_934a9/1 -> Divide_d9d2a/1
  Power_d7519/1 -> Divide_d9d2a/2
  Subtract_56b16/1 -> Divide_e738d/1
  Constant_x_ddd_caf9c/1 -> Divide_e738d/2
  Constant_x_d_b5ef4/1 -> Subtract_1b8ec/1
  Constant_x_dd_8482f/1 -> Subtract_1b8ec/2
  Divide_d9d2a/1 -> Subtract_2704a/1
  Divide_e738d/1 -> Subtract_2704a/2
  State_psi_fd_SG_D_13_37be0/1 -> Subtract_c4390/2
  Subtract_2704a/1 -> Product_a5637/2
  Subtract_c4390/1 -> Subtract_7c9b3/1
  Product_a5637/1 -> Subtract_7c9b3/2
  Subtract_7c9b3/1 -> Divide_505fe/1
  Constant_T_dd_788cd/1 -> Divide_505fe/2
  Divide_505fe/1 -> Blockout_d_psi_fd_SG_D_13_87f69/1

== system IEEE30_case/SG_D_13/d_psi_gq_SG_D_13_block ==
  note: d_psi_gq_SG_D_13 in IEEE30_case
      | $-\frac{\psi _{\mathrm{gq},\mathrm{SG},D,13}+\left(x_{q}-x_{\mathrm{qd}}\right)\,\left(\frac{\psi _{q,\mathrm{SG},D,13}+\frac{\psi _{\mathrm{gq},\mathrm{SG},D,13}\,\left(x_{l}-x_{\mathrm{qdd}}\right)}{x_{l}-x_{\mathrm{qd}}}+\frac{\psi _{\mathrm{kq},\mathrm{SG},D,13}\,\left(x_{\mathrm{qd}}-x_{\mathrm{qdd}}\right)}{x_{l}-x_{\mathrm{qd}}}}{x_{\mathrm{qdd}}}+\frac{\left(x_{\mathrm{qd}}-x_{\mathrm{qdd}}\right)\,\left(\psi _{\mathrm{gq},\mathrm{SG},D,13}+\psi _{\mathrm{kq},\mathrm{SG},D,13}+\frac{\left(x_{l}-x_{\mathrm{qd}}\right)\,\left(\psi _{q,\mathrm{SG},D,13}+\frac{\psi _{\mathrm{gq},\mathrm{SG},D,13}\,\left(x_{l}-x_{\mathrm{qdd}}\right)}{x_{l}-x_{\mathrm{qd}}}+\frac{\psi _{\mathrm{kq},\mathrm{SG},D,13}\,\left(x_{\mathrm{qd}}-x_{\mathrm{qdd}}\right)}{x_{l}-x_{\mathrm{qd}}}\right)}{x_{\mathrm{qdd}}}\right)}{{\left(x_{l}-x_{\mathrm{qd}}\right)}^2}\right)}{T_{\mathrm{qd}}}$
      | Automatically generated on 2025-11-01 18:34:59 .
  State_psi_gq_SG_D_13_d26d2 : Inport
  State_psi_gq_SG_D_13_12a06 : Inport  Port=2
  State_psi_kq_SG_D_13_0827f : Inport  Port=3
  State_psi_gq_SG_D_13_9dfd7 : Inport  Port=4
  State_psi_kq_SG_D_13_78acb : Inport  Port=5
  State_psi_q_SG_D_13_40583 : Inport  Port=6
  State_psi_gq_SG_D_13_f8d15 : Inport  Port=7
  State_psi_kq_SG_D_13_7423f : Inport  Port=8
  State_psi_q_SG_D_13_9a89d : Inport  Port=9
  Add_35426 : Sum
  Add_36262 : Sum
  Add_5873c : Sum
  Add_5ab34 : Sum
  Add_5d16f : Sum
  Add_87136 : Sum
  Add_902c2 : Sum
  Add_a8e28 : Sum
  Add_aa27f : Sum
  Add_b4cbe : Sum
  Add_b9cd8 : Sum
  Add_d43bf : Sum
  Constant_-1_07699 : Constant  Value=-1
  Constant_-1_19c92 : Constant  Value=-1
  Constant_-1_1b249 : Constant  Value=-1
  Constant_-1_2dc94 : Constant  Value=-1
  Constant_-1_4d100 : Constant  Value=-1
  Constant_-1_54088 : Constant  Value=-1
  Constant_-1_6c348 : Constant  Value=-1
  Constant_-1_988e4 : Constant  Value=-1
  Constant_-1_a9dd9 : Constant  Value=-1
  Constant_-1_c7a6b : Constant  Value=-1
  Constant_2.0_d3c02 : Constant  Value=2.0
  Constant_T_qd_6827b : Constant  Value=T_qd
  Constant_x_l_0dae2 : Constant  Value=x_l
  Constant_x_l_40861 : Constant  Value=x_l
  Constant_x_l_6d292 : Constant  Value=x_l
  Constant_x_l_a281a : Constant  Value=x_l
  Constant_x_l_b98b8 : Constant  Value=x_l
  Constant_x_l_cd2a4 : Constant  Value=x_l
  Constant_x_l_ce2a8 : Constant  Value=x_l
  Constant_x_l_f1726 : Constant  Value=x_l
  Constant_x_q_2a484 : Constant  Value=x_q
  Constant_x_qd_093fc : Constant  Value=x_qd
  Constant_x_qd_1a4fc : Constant  Value=x_qd
  Constant_x_qd_23a3e : Constant  Value=x_qd
  Constant_x_qd_2d300 : Constant  Value=x_qd
  Constant_x_qd_79022 : Constant  Value=x_qd
  Constant_x_qd_8b06a : Constant  Value=x_qd
  Constant_x_qd_b511f : Constant  Value=x_qd
  Constant_x_qd_e653b : Constant  Value=x_qd
  Constant_x_qd_ee6c2 : Constant  Value=x_qd
  Constant_x_qd_f2d2b : Constant  Value=x_qd
  Constant_x_qdd_0e03d : Constant  Value=x_qdd
  Constant_x_qdd_1a396 : Constant  Value=x_qdd
  Constant_x_qdd_53013 : Constant  Value=x_qdd
  Constant_x_qdd_5a83b : Constant  Value=x_qdd
  Constant_x_qdd_5b249 : Constant  Value=x_qdd
  Constant_x_qdd_94729 : Constant  Value=x_qdd
  Constant_x_qdd_f26e2 : Constant  Value=x_qdd
  Divide_02084 : Product  Inputs=*/
  Divide_222dd : Product  Inputs=*/
  Divide_3b936 : Product  Inputs=*/
  Divide_81fc8 : Product  Inputs=*/
  Divide_89101 : Product  Inputs=*/
  Divide_8a893 : Product  Inputs=*/
  Divide_99821 : Product  Inputs=*/
  Divide_a0f55 : Product  Inputs=*/
  Power_ef981 : Math  Operator=pow
  Product_0ac7b : Product
  Product_29ebb : Product
  Product_38c34 : Product
  Product_3dda3 : Product
  Product_4f9fe : Product
  Product_76c74 : Product
  Product_78368 : Product
  Product_7e440 : Product
  Product_85126 : Product
  Product_91bf8 : Product
  Product_9977b : Product
  Product_a172a : Product
  Product_bf400 : Product
  Product_e1d81 : Product
  Product_e2873 : Product
  Product_e7da8 : Product
  Product_ea558 : Product
  Subtract_1be7a : Sum  Inputs=+-
  Subtract_1f642 : Sum  Inputs=+-
  Subtract_2be4e : Sum  Inputs=+-
  Subtract_653a0 : Sum  Inputs=+-
  Subtract_7bb85 : Sum  Inputs=+-
  Subtract_c82b5 : Sum  Inputs=+-
  Subtract_f2944 : Sum  Inputs=+-
  Subtract_fd608 : Sum  Inputs=+-
  Blockout_d_psi_gq_SG_D_13_d3799 : Outport
  wires:
  Constant_x_qdd_5a83b/1 -> Add_87136/2
  Constant_-1_1b249/1 -> Product_4f9fe/1
  Product_4f9fe/1 -> Add_87136/1
  Subtract_1be7a/1 -> Add_5ab34/1
  Constant_x_l_ce2a8/1 -> Product_4f9fe/2
  Constant_x_qd_e653b/1 -> Add_d43bf/2
  Constant_x_l_b98b8/1 -> Product_7e440/2
  Product_bf400/1 -> Add_35426/1
  Constant_-1_54088/1 -> Product_bf400/1
  Subtract_653a0/1 -> Product_a172a/2
  Constant_x_qd_79022/1 -> Subtract_653a0/1
  Constant_x_l_6d292/1 -> Product_bf400/2
  Add_902c2/1 -> Divide_99821/2
  Constant_x_qdd_0e03d/1 -> Subtract_653a0/2
  Product_76c74/1 -> Add_902c2/1
  Constant_-1_4d100/1 -> Product_76c74/1
  Constant_x_l_0dae2/1 -> Product_76c74/2
  Product_29ebb/1 -> Divide_81fc8/1
  State_psi_gq_SG_D_13_9dfd7/1 -> Product_29ebb/1
  Add_87136/1 -> Product_29ebb/2
  Constant_x_qd_8b06a/1 -> Add_35426/2
  Product_a172a/1 -> Divide_99821/1
  State_psi_kq_SG_D_13_78acb/1 -> Product_a172a/1
  Constant_x_qd_ee6c2/1 -> Add_902c2/2
  Constant_x_l_a281a/1 -> Product_e2873/2
  Add_35426/1 -> Divide_81fc8/2
  Product_7e440/1 -> Add_b9cd8/1
  Constant_-1_a9dd9/1 -> Product_7e440/1
  Divide_81fc8/1 -> Subtract_1be7a/1
  State_psi_q_SG_D_13_40583/1 -> Add_5ab34/2
  Divide_99821/1 -> Subtract_1be7a/2
  Product_85126/1 -> Add_36262/1
  Constant_-1_6c348/1 -> Product_85126/1
  Add_d43bf/1 -> Divide_8a893/2
  Product_78368/1 -> Divide_02084/1
  Constant_x_l_f1726/1 -> Product_85126/2
  Constant_x_qd_23a3e/1 -> Add_b9cd8/2
  Product_e2873/1 -> Add_d43bf/1
  Add_b9cd8/1 -> Product_78368/1
  Constant_-1_19c92/1 -> Product_e2873/1
  Constant_x_qdd_5b249/1 -> Add_36262/2
  Constant_-1_2dc94/1 -> Product_9977b/1
  Product_0ac7b/1 -> Add_aa27f/1
  Constant_-1_07699/1 -> Product_0ac7b/1
  Subtract_f2944/1 -> Product_91bf8/2
  Constant_x_qd_1a4fc/1 -> Subtract_f2944/1
  Constant_x_l_40861/1 -> Product_0ac7b/2
  Constant_x_qdd_1a396/1 -> Subtract_f2944/2
  Add_5ab34/1 -> Product_78368/2
  Product_3dda3/1 -> Divide_222dd/1
  State_psi_gq_SG_D_13_f8d15/1 -> Product_3dda3/1
  Add_36262/1 -> Product_3dda3/2
  Constant_x_qd_2d300/1 -> Add_aa27f/2
  Product_91bf8/1 -> Divide_8a893/1
  Constant_x_qdd_94729/1 -> Subtract_2be4e/2
  Subtract_7bb85/1 -> Product_e7da8/2
  State_psi_kq_SG_D_13_7423f/1 -> Product_91bf8/1
  Subtract_2be4e/1 -> Product_9977b/2
  Constant_x_qd_f2d2b/1 -> Subtract_2be4e/1
  State_psi_gq_SG_D_13_12a06/1 -> Add_5d16f/1
  State_psi_kq_SG_D_13_0827f/1 -> Add_5d16f/2
  Constant_x_qdd_f26e2/1 -> Divide_02084/2
  Constant_-1_988e4/1 -> Product_ea558/1
  Constant_x_l_cd2a4/1 -> Product_ea558/2
  Add_aa27f/1 -> Divide_222dd/2
  Add_5d16f/1 -> Subtract_7bb85/1
  Divide_02084/1 -> Subtract_7bb85/2
  Product_ea558/1 -> Add_b4cbe/1
  Constant_x_qd_b511f/1 -> Add_b4cbe/2
  Divide_222dd/1 -> Subtract_c82b5/1
  Divide_8a893/1 -> Subtract_c82b5/2
  Product_9977b/1 -> Product_e7da8/1
  Add_b4cbe/1 -> Power_ef981/1
  Constant_2.0_d3c02/1 -> Power_ef981/2
  Subtract_c82b5/1 -> Add_5873c/1
  State_psi_q_SG_D_13_9a89d/1 -> Add_5873c/2
  Constant_-1_c7a6b/1 -> Product_38c34/1
  Product_e7da8/1 -> Divide_3b936/1
  Power_ef981/1 -> Divide_3b936/2
  Add_5873c/1 -> Divide_a0f55/1
  Constant_x_qdd_53013/1 -> Divide_a0f55/2
  Constant_x_q_2a484/1 -> Subtract_1f642/1
  Constant_x_qd_093fc/1 -> Subtract_1f642/2
  Divide_3b936/1 -> Subtract_fd608/1
  Divide_a0f55/1 -> Subtract_fd608/2
  State_psi_gq_SG_D_13_d26d2/1 -> Product_38c34/2
  Subtract_1f642/1 -> Product_e1d81/1
  Subtract_fd608/1 -> Product_e1d81/2
  Product_38c34/1 -> Add_a8e28/1
  Product_e1d81/1 -> Add_a8e28/2
  Add_a8e28/1 -> Divide_89101/1
  Constant_T_qd_6827b/1 -> Divide_89101/2
  Divide_89101/1 -> Blockout_d_psi_gq_SG_D_13_d3799/1

== system IEEE30_case/SG_D_13/d_psi_kq_SG_D_13_block ==
  note: d_psi_kq_SG_D_13 in IEEE30_case
      | $-\frac{\psi _{\mathrm{gq},\mathrm{SG},D,13}+\psi _{\mathrm{kq},\mathrm{SG},D,13}+\frac{\left(x_{l}-x_{\mathrm{qd}}\right)\,\left(\psi _{q,\mathrm{SG},D,13}+\frac{\psi _{\mathrm{gq},\mathrm{SG},D,13}\,\left(x_{l}-x_{\mathrm{qdd}}\right)}{x_{l}-x_{\mathrm{qd}}}+\frac{\psi _{\mathrm{kq},\mathrm{SG},D,13}\,\left(x_{\mathrm{qd}}-x_{\mathrm{qdd}}\right)}{x_{l}-x_{\mathrm{qd}}}\right)}{x_{\mathrm{qdd}}}}{T_{\mathrm{qdd}}}$
      | Automatically generated on 2025-11-01 18:35:02 .
  State_psi_gq_SG_D_13_cdb7e : Inport
  State_psi_kq_SG_D_13_cfe97 : Inport  Port=2
  State_psi_gq_SG_D_13_0b0ed : Inport  Port=3
  State_psi_kq_SG_D_13_80acc : Inport  Port=4
  State_psi_q_SG_D_13_4239b : Inport  Port=5
  Add_3ea33 : Sum
  Add_6afd0 : Sum
  Add_98c4c : Sum
  Add_b3622 : Sum
  Add_d608e : Sum
  Add_ea8ea : Sum
  Constant_-1_1d0ef : Constant  Value=-1
  Constant_-1_368b9 : Constant  Value=-1
  Constant_-1_759c0 : Constant  Value=-1
  Constant_-1_bc692 : Constant  Value=-1
  Constant_-1_f00f1 : Constant  Value=-1
  Constant_T_qdd_e4cc6 : Constant  Value=T_qdd
  Constant_x_l_45097 : Constant  Value=x_l
  Constant_x_l_561c7 : Constant  Value=x_l
  Constant_x_l_80081 : Constant  Value=x_l
  Constant_x_l_9c3e6 : Constant  Value=x_l
  Constant_x_qd_1f69d : Constant  Value=x_qd
  Constant_x_qd_5737e : Constant  Value=x_qd
  Constant_x_qd_5ae49 : Constant  Value=x_qd
  Constant_x_qd_e4240 : Constant  Value=x_qd
  Constant_x_qdd_b64cd : Constant  Value=x_qdd
  Constant_x_qdd_ceaa9 : Constant  Value=x_qdd
  Constant_x_qdd_dd327 : Constant  Value=x_qdd
  Divide_bf92d : Product  Inputs=*/
  Divide_c18bd : Product  Inputs=*/
  Divide_cf08b : Product  Inputs=*/
  Divide_ddc13 : Product  Inputs=*/
  Product_4919e : Product
  Product_63058 : Product
  Product_7210f : Product
  Product_99334 : Product
  Product_bbec3 : Product
  Product_c9b09 : Product
  Product_d05f9 : Product
  Product_e7eca : Product
  Subtract_6ea58 : Sum  Inputs=+-
  Subtract_72227 : Sum  Inputs=+-
  Subtract_be032 : Sum  Inputs=+-
  Blockout_d_psi_kq_SG_D_13_a0846 : Outport
  wires:
  Product_c9b09/1 -> Add_6afd0/1
  Product_4919e/1 -> Add_ea8ea/1
  Constant_-1_759c0/1 -> Product_4919e/1
  Divide_cf08b/1 -> Subtract_6ea58/1
  Constant_-1_368b9/1 -> Product_d05f9/1
  Product_bbec3/1 -> Add_98c4c/1
  Constant_-1_f00f1/1 -> Product_bbec3/1
  Constant_x_l_45097/1 -> Product_4919e/2
  Constant_x_qdd_ceaa9/1 -> Add_d608e/2
  Product_d05f9/1 -> Add_d608e/1
  Add_b3622/1 -> Divide_ddc13/1
  Constant_x_l_561c7/1 -> Product_d05f9/2
  Subtract_be032/1 -> Product_7210f/2
  Constant_x_qd_1f69d/1 -> Subtract_be032/1
  Constant_x_qdd_b64cd/1 -> Subtract_be032/2
  Add_6afd0/1 -> Product_e7eca/1
  Constant_x_l_9c3e6/1 -> Product_bbec3/2
  Subtract_72227/1 -> Add_b3622/1
  State_psi_gq_SG_D_13_0b0ed/1 -> Product_99334/1
  Add_d608e/1 -> Product_99334/2
  Constant_x_qd_5737e/1 -> Add_ea8ea/2
  Product_7210f/1 -> Divide_bf92d/1
  State_psi_kq_SG_D_13_80acc/1 -> Product_7210f/1
  Add_ea8ea/1 -> Divide_cf08b/2
  Constant_x_qd_5ae49/1 -> Add_98c4c/2
  Product_99334/1 -> Divide_cf08b/1
  Add_98c4c/1 -> Divide_bf92d/2
  Constant_-1_bc692/1 -> Product_c9b09/1
  Constant_x_l_80081/1 -> Product_c9b09/2
  Divide_bf92d/1 -> Subtract_6ea58/2
  Constant_x_qd_e4240/1 -> Add_6afd0/2
  Subtract_6ea58/1 -> Add_3ea33/1
  Product_63058/1 -> Subtract_72227/1
  Add_3ea33/1 -> Product_e7eca/2
  State_psi_q_SG_D_13_4239b/1 -> Add_3ea33/2
  Constant_-1_1d0ef/1 -> Product_63058/1
  State_psi_gq_SG_D_13_cdb7e/1 -> Product_63058/2
  State_psi_kq_SG_D_13_cfe97/1 -> Subtract_72227/2
  Product_e7eca/1 -> Divide_c18bd/1
  Constant_x_qdd_dd327/1 -> Divide_c18bd/2
  Divide_c18bd/1 -> Add_b3622/2
  Constant_T_qdd_e4cc6/1 -> Divide_ddc13/2
  Divide_ddc13/1 -> Blockout_d_psi_kq_SG_D_13_a0846/1
